simulink model "Case_SG_Simulation_v2"  (R2020b)
settings: Solver=FixedStepAuto  StartTime=0  StopTime=20  FixedStep=Ts  RelTol=1e-3
undefined symbols (not defined in the file or in its folder): DeviceDiscreDamping, DevicePara, DeviceType, OtherInputs, PowerFlow, Ts, Wbase, x_e, Zbase
libraries: powerlib x6, Simplex_PowerSystems x6
settings Model: Creator=admin_user  LastModifiedBy=admin_user
settings DataIOCC: ReturnWorkspaceOutputs=off

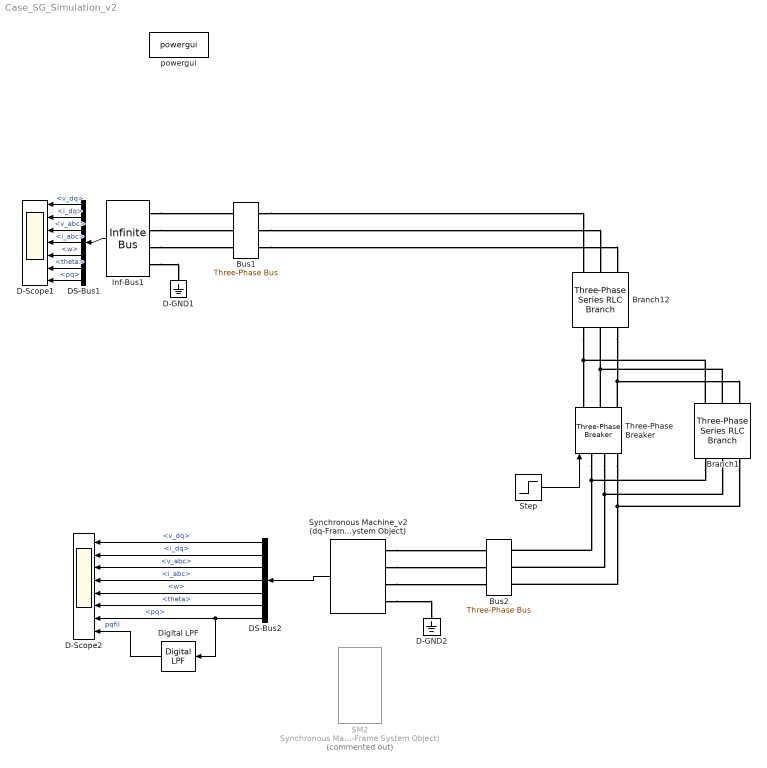
== system Case_SG_Simulation_v2 ==
  Branch1 : powerlib/Elements/Three-Phase Series RLC Branch  LConnTagsString=A|B|C  RConnTagsString=A|B|C  BranchType=R  Resistance=0.3*Zbase  Inductance=(0.65)*Zbase/Wbase  Capacitance=1e-6  Measurements=None
  Branch12 : powerlib/Elements/Three-Phase Series RLC Branch  LConnTagsString=A|B|C  RConnTagsString=A|B|C  BranchType=L  Resistance=(0)*Zbase  Inductance=(0.65)*Zbase/Wbase  Capacitance=1e-6  Measurements=None
  Bus1 : Simplex_PowerSystems/Three-Phase Bus  Vbase=1  Sbase=1
      settings: SourceProductName=Simplex Power Systems
  Bus2 : Simplex_PowerSystems/Three-Phase Bus  Vbase=1  Sbase=1
      settings: SourceProductName=Simplex Power Systems
  D-GND1 : powerlib/Elements/Ground  LConnTagsString=a
  D-GND2 : powerlib/Elements/Ground  LConnTagsString=a
  D-Scope1 : Scope  NumInputPorts=7
  D-Scope2 : Scope  NumInputPorts=8
  DS-Bus1 : BusSelector  OutputSignals=v_dq,i_dq,v_abc,i_abc,w,theta,pq
  DS-Bus2 : BusSelector  OutputSignals=v_dq,i_dq,v_abc,i_abc,w,theta,pq
  Digital LPF : Simplex_PowerSystems/Digital LPF  wfil=5*2*pi  Ts=Ts
      settings: SourceProductName=Simplex Power Systems
  Inf-Bus1 : Simplex_PowerSystems/Infinite Bus  Sbase=Sbase  Vbase=Vbase  Wbase=Wbase  vd=1  vq=0  theta0=0  w=Wbase  Ts=Ts  R=1e-30
      settings: SourceProductName=Simplex Power Systems
  SM2 : Simplex_PowerSystems/Synchronous Machine (dq-Frame System Object)  Commented=on  Sbase=Sbase  Vbase=Vbase  Wbase=Wbase  DeviceType=DeviceType{2}  DevicePara=DevicePara{2}  PowerFlow=PowerFlow{2}  x0=x_e{2}  OtherInputs=OtherInputs{2}  Ts=Ts  DiscreMethod=Hybrid Trapezoidal  EnableInsideModification=off  DiscreDampingFlag=on  DiscreDampingValue=DeviceDiscreDamping{2}  LinearizationTimes=1  DirectFeedthrough=off
      settings: SourceProductName=Simplex Power Systems
  Step : Step  Time=10  Before=1  After=0  SampleTime=0
  Synchronous Machine_v2 (dq-Frame System Object) : Simplex_PowerSystems/Synchronous Machine_v2 (dq-Frame System Object)  Sbase=Sbase  Vbase=Vbase  Wbase=Wbase  DeviceType=DeviceType{2}  DevicePara=DevicePara{2}  PowerFlow=PowerFlow{2}  x0=x_e{2}  OtherInputs=OtherInputs{2}  Ts=Ts  DiscreMethod=Hybrid Trapezoidal  EnableInsideModification=off  DiscreDampingFlag=on  DiscreDampingValue=DeviceDiscreDamping{2}  LinearizationTimes=1  DirectFeedthrough=off
      settings: SourceProductName=Simplex Power Systems
  Three-Phase Breaker : powerlib/Elements/Three-Phase Breaker  InitialState=closed  SwitchA=on  SwitchB=on  SwitchC=on  SwitchTimes="[1/60  5/60]"  External=on  BreakerResistance=0.01  SnubberResistance=1e6  SnubberCapacitance=inf  Measurements=None
  powergui : powerlib/powergui  Priority=1  SimulationMode=Discrete  SampleTime=Ts  frequency=60  Iterations=50  frequencyindice=0  Pbase=100e6  ErrMax=1e-4  UnitsV=kV  UnitsW=MW  buscounter=0  FunctionMessages=off  echomessages=off  EnableUseOfTLC=off  CurrentSourceSwitches=off  DisableSnubberDevices=off  DisableRonSwitches=off  DisableVfSwitches=off  DisplayEquations=off  AutomaticDiscreteSolvers=off  SolverType=Tustin/Backward Euler (TBE)  Interpol=off  ExternalGateDelay=off  methode=off  Ts=100  x0status=blocks  SPID=on  SwTol=0  HookPort=off  NonlinearTolerance=1e-4  nMaxIteration=100  ContinueOnMaxIteration=off  RestoreLinks=warning  ResistiveCurrentMeasurement=off  Frange=[0:2:500]  Ylog=off  Xlog=on  ShowGrid=off  save=off  variable=ZData  structure=0  ZoomFFT=off  StartTime=0.0  cycles=1  DisplayStyle=1  fundamental=60  FreqAxis=off  MaxFrequency=1000  frequencyindicesteady=1  RmsSteady=1  display=off
  wires:
  Inf-Bus1/1 -> DS-Bus1/1
  DS-Bus1/1 -> D-Scope1/1  "<v_dq>"
  DS-Bus1/2 -> D-Scope1/2  "<i_dq>"
  DS-Bus1/3 -> D-Scope1/3  "<v_abc>"
  DS-Bus1/4 -> D-Scope1/4  "<i_abc>"
  DS-Bus1/5 -> D-Scope1/5  "<w>"
  DS-Bus1/6 -> D-Scope1/6  "<theta>"
  DS-Bus1/7 -> D-Scope1/7  "<pq>"
  Synchronous Machine_v2 (dq-Frame System Object)/1 -> DS-Bus2/1
  DS-Bus2/1 -> D-Scope2/1  "<v_dq>"
  DS-Bus2/2 -> D-Scope2/2  "<i_dq>"
  DS-Bus2/3 -> D-Scope2/3  "<v_abc>"
  DS-Bus2/4 -> D-Scope2/4  "<i_abc>"
  DS-Bus2/5 -> D-Scope2/5  "<w>"
  DS-Bus2/6 -> D-Scope2/6  "<theta>"
  DS-Bus2/7 -> Digital LPF/1, D-Scope2/7  "<pq>"
  Step/1 -> Three-Phase Breaker/1
  Digital LPF/1 -> D-Scope2/8  "pqfil"
  connections:
  Inf-Bus1/LConn1 -- Bus1/LConn1
  Inf-Bus1/LConn2 -- Bus1/LConn2
  Inf-Bus1/LConn3 -- Bus1/LConn3
  Synchronous Machine_v2 (dq-Frame System Object)/LConn1 -- Bus2/LConn1
  Synchronous Machine_v2 (dq-Frame System Object)/LConn2 -- Bus2/LConn2
  Synchronous Machine_v2 (dq-Frame System Object)/LConn3 -- Bus2/LConn3
  Inf-Bus1/LConn4 -- D-GND1/LConn1
  Synchronous Machine_v2 (dq-Frame System Object)/LConn4 -- D-GND2/LConn1
  Bus1/RConn1 -- Branch12/LConn1
  Bus1/RConn2 -- Branch12/LConn2
  Bus1/RConn3 -- Branch12/LConn3
  Branch12/RConn1 -- Branch1/LConn1 -- Three-Phase Breaker/RConn1
  Three-Phase Breaker/RConn2 -- Branch1/LConn2 -- Branch12/RConn2
  Three-Phase Breaker/RConn3 -- Branch12/RConn3 -- Branch1/LConn3
  Three-Phase Breaker/LConn1 -- Branch1/RConn1 -- Bus2/RConn1
  Three-Phase Breaker/LConn2 -- Branch1/RConn2 -- Bus2/RConn2
  Three-Phase Breaker/LConn3 -- Branch1/RConn3 -- Bus2/RConn3
